simulink model "main2"  (R2024a)
settings: Solver=ode15s  StartTime=0.0  StopTime=2  MaxStep=1e-4  RelTol=1e-3
InitFcn:
  | parametros
values from neighbouring files (symbols this model uses):
  alpha_cu = 3.9 *10^-3    (= 0.0039)    [parametros.m]
  b_l = 0.1    [parametros.m]
  b_m = 1.5 * 10^-5    (= 1.5e-05)    [parametros.m]
  C_ts = 0.818    [parametros.m]
  J_l = (m*l_cm^2 + J_cm) + (m_l * l_l^2)    (= 0.0833)    [parametros.m]
  J_m = 1.4 * 10^-5    (= 1.4e-05)    [parametros.m]
  k_l = m * g * l_cm + m_l * g * l_l    (= 2.4516625)    [parametros.m]
  L_d = 6.6 * 10^-3    (= 0.0066)    [parametros.m]
  L_ls = 0.8 * 10^-3    (= 0.0008)    [parametros.m]
  L_q = 5.8 * 10^-3    (= 0.0058)    [parametros.m]
  lambda_m = 0.016    [parametros.m]
  P_p = 3    [parametros.m]
  r = 120    [parametros.m]
  R_s_40 = 1.02    [parametros.m]
  R_ts_amb = 146.7    [parametros.m]
  Temp_s_ref = 40    [parametros.m]
undefined symbols (not defined in the file or in its folder): K_e_omega, K_e_theta
libraries: simulink x6
(part 1 of 2)
settings Model: Creator=Usuario  LastModifiedBy=Usuario

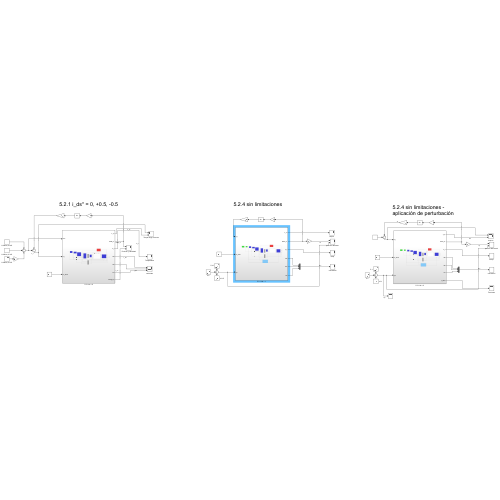
[thumbnail: Simulink's stored preview of the top-level diagram]
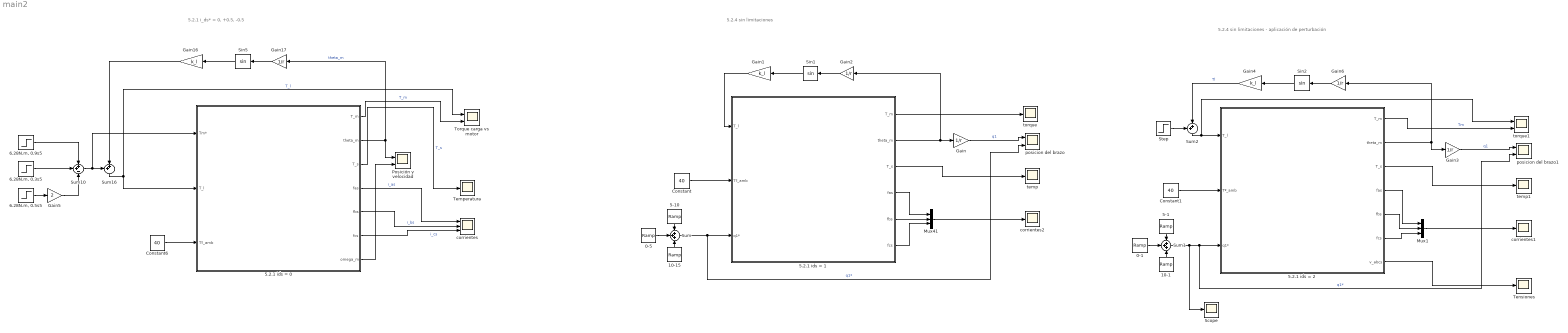
== system main2 ==
  note: 5.2.1 i_ds* = 0, +0.5, -0.5
  note: 5.2.4 sin limitaciones
  note: 5.2.4 sin limitaciones - aplicación de perturbación
  0-1 : simulink/Sources/Ramp  slope=1/5  start=0  InitialOutput=0
  0-5 : simulink/Sources/Ramp  slope=2*pi/5  start=0  InitialOutput=0
  10-1 : simulink/Sources/Ramp  slope=-1/5  start=10  InitialOutput=0
  10-15 : simulink/Sources/Ramp  slope=-2*pi/5  start=10  InitialOutput=0
  5-1 : simulink/Sources/Ramp  slope=-1/5  start=5  InitialOutput=0
  5-10 : simulink/Sources/Ramp  slope=-2*pi/5  start=5  InitialOutput=0
  5.2.1 ids = 0 : Subsystem
  5.2.1 ids = 1 : Subsystem
  5.2.1 ids = 2 : Subsystem
  "6.28N.m, 0.3s5" : Step  Time=0.3  After=6.28  SampleTime=0
  "6.28N.m, 0.5s5" : Step  Time=.5  After=6.28  SampleTime=0
  "6.28N.m, 0.9s5" : Step  Time=.9  After=6.28  SampleTime=0
  Constant : Constant  Value=40
  Constant1 : Constant  Value=40
  Constant6 : Constant  Value=40
  Gain{,2..3,6,17} (5 alike) : Gain  Gain=1/r
  Gain1 : Gain  Gain=k_l
  Gain16 : Gain  Gain=k_l
  Gain4 : Gain  Gain=k_l
  Gain5 : Gain  Gain=2
  Mux1 : Mux  Inputs=3
  Mux41 : Mux  Inputs=3
  Posición y velocidad : Scope  NumInputPorts=2
  Scope : Scope
  Sin1 : Trigonometry
  Sin2 : Trigonometry
  Sin5 : Trigonometry
  Step : Step  Time=7.5  After=2*pi  SampleTime=0
  Sum : Sum  Inputs=+++
  Sum1 : Sum  Inputs=+++
  Sum10 : Sum  Inputs=++-
  Sum16 : Sum  Inputs=++|
  Sum2 : Sum  Inputs=++|
  Temperatura : Scope
  Tensiones : Scope
  Torque carga vs motor : Scope  NumInputPorts=2
  corrientes : Scope  NumInputPorts=3
  corrientes1 : Scope
  corrientes2 : Scope
  posicion del brazo : Scope  NumInputPorts=2
  posicion del brazo1 : Scope  NumInputPorts=2
  temp : Scope
  temp1 : Scope
  torque : Scope
  torque1 : Scope  NumInputPorts=2
  wires:
  5.2.1 ids = 1/6(fcs) -> Mux41/3
  5.2.1 ids = 1/4(fas) -> Mux41/1
  5.2.1 ids = 1/5(fbs) -> Mux41/2
  Mux41/1 -> corrientes2/1
  5.2.1 ids = 1/2("theta_m ") -> Gain/1, Gain2/1
  Sin1/1 -> Gain1/1
  Gain2/1 -> Sin1/1
  Constant/1 -> 5.2.1 ids = 1/2(Tº_amb)
  5.2.1 ids = 1/3(T_s) -> temp/1
  "6.28N.m, 0.3s5"/1 -> Sum10/2
  5.2.1 ids = 0/2("theta_m ") -> Posición y velocidad/1, Gain17/1  "theta_m"
  Constant6/1 -> 5.2.1 ids = 0/3(Tº_amb)
  "6.28N.m, 0.5s5"/1 -> Gain5/1
  Gain5/1 -> Sum10/3
  5.2.1 ids = 0/6(fcs) -> corrientes/3  "i_cs"
  5.2.1 ids = 0/5(fbs) -> corrientes/2  "i_bs"
  5.2.1 ids = 0/1(T_m) -> Torque carga vs motor/2  "T_m"
  5.2.1 ids = 0/4(fas) -> corrientes/1  "i_as"
  Sum16/1 -> 5.2.1 ids = 0/2(T_l), Torque carga vs motor/1  "T_l"
  5.2.1 ids = 0/3(T_s) -> Temperatura/1  "T_s"
  Gain17/1 -> Sin5/1
  "6.28N.m, 0.9s5"/1 -> Sum10/1
  Sin5/1 -> Gain16/1
  5.2.1 ids = 1/1(T_m) -> torque/1
  Gain1/1 -> 5.2.1 ids = 1/1(T_l)
  Sum/1 -> posicion del brazo/2, 5.2.1 ids = 1/3(q1*)  "q1*"
  0-5/1 -> Sum/2
  Gain/1 -> posicion del brazo/1  "q1"
  5-10/1 -> Sum/1
  10-15/1 -> Sum/3
  5-1/1 -> Sum1/1
  Sum1/1 -> Scope/1, posicion del brazo1/2, 5.2.1 ids = 2/3(q1*)  "q1*"
  0-1/1 -> Sum1/2
  5.2.1 ids = 2/1(T_m) -> torque1/2  "Tm"
  Gain3/1 -> posicion del brazo1/1  "q1"
  10-1/1 -> Sum1/3
  Mux1/1 -> corrientes1/1
  5.2.1 ids = 2/3(T_s) -> temp1/1
  5.2.1 ids = 2/6(fcs) -> Mux1/3
  5.2.1 ids = 2/5(fbs) -> Mux1/2
  Constant1/1 -> 5.2.1 ids = 2/2(Tº_amb)
  Gain6/1 -> Sin2/1
  5.2.1 ids = 2/2("theta_m ") -> Gain3/1, Gain6/1
  5.2.1 ids = 2/4(fas) -> Mux1/1
  Sin2/1 -> Gain4/1
  Gain4/1 -> Sum2/2  "Tl"
  Sum2/1 -> torque1/1, 5.2.1 ids = 2/1(T_l)
  Step/1 -> Sum2/1
  5.2.1 ids = 2/7(v_abcs) -> Tensiones/1
  Gain16/1 -> Sum16/2
  Sum10/1 -> 5.2.1 ids = 0/1(Tm*), Sum16/1
  5.2.1 ids = 0/7(omega_m) -> Posición y velocidad/2

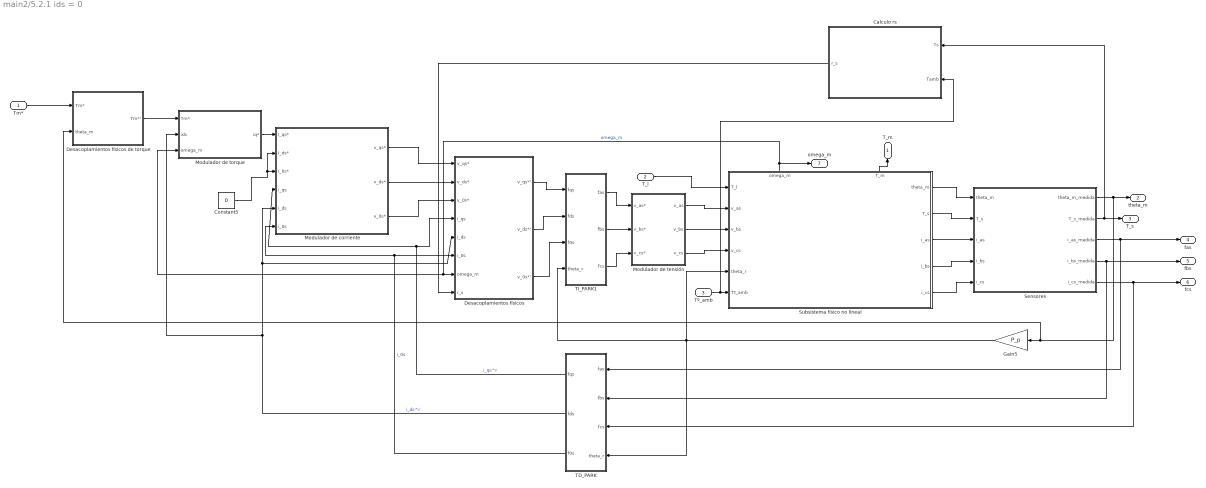
== system main2/5.2.1 ids = 0 ==
  Tm* : Inport
  T_l : Inport  Port=2
  Tº_amb : Inport  Port=3
  Calculo rs : Subsystem
  Constant5 : Constant  Value=0
  Desacoplamientos físicos : Subsystem
  Desacoplamientos físicos de torque : Subsystem
  Gain5 : Gain  Gain=P_p
  Modulador de corriente : Subsystem
  Modulador de tensión : Subsystem
  Modulador de torque : Subsystem
  Sensores : Subsystem
  "Subsistema físico no lineal " : Subsystem
      settings: PortSchema="{\"entries\":[{\"content\":{\"sides\":[{\"content\":{\"connectorIds\":[\"In1\",\"In2\",\"In3\",\"In4\",\"In5\",\"In6\"]},\"type\":\"ConnectorPlacement.EquallySpacedRectSide\",\"uuid\":\"df16c937-5b0d-437b-9581-4e7e4443d731\"},{\"content\":{\"connectorIds\":[\"Out1\",\"Out2\",\"Out3\",\"Out4\",\"Out5\"],\"side\":\"RIGHT\"},\"type\":\"ConnectorPlacement.EquallySpacedRectSide\",\"uuid\":\"58799b56-1bb2-4861-ad63-3fa3f8181ad5\"},{\"content\":{\"connectorIds\":[\"Out6\",\"Out7\"],\"side\":\"TOP\"},\"type\":\"ConnectorPlacement.EquallySpacedRectSide\",\"uuid\":\"9d658df7-49d2-4fa1-a84c-b158d9dac98e\"}]},\"type\":\"ConnectorPlacement.EquallySpacedConnector\",\"uuid\":\"4e139d46-6a94-417e-9cad-9c9676c83a39\"}],\"packageUris\":[\"http://schema.mathworks.com/mf0/Connector/R2020b\"],\"version\":\"1.0\"}"
  TD_PARK : MATLAB Function  TreatAsAtomicUnit=on
  TI_PARK1 : MATLAB Function  TreatAsAtomicUnit=on
  T_m : Outport
  "theta_m " : Outport  Port=2
  T_s : Outport  Port=3
  fas : Outport  Port=4
  fbs : Outport  Port=5
  fcs : Outport  Port=6
  omega_m : Outport  Port=7
  wires:
  Modulador de tensión/1(v_as) -> "Subsistema físico no lineal "/2(v_as)
  TD_PARK/3(f0s) -> Desacoplamientos físicos/6(i_0s), Modulador de corriente/6(i_0s)  "i_0s"
  TI_PARK1/1(fas) -> Modulador de tensión/1(v_as*)
  Sensores/2(T_s_medida) -> T_s/1, Calculo rs/1(Ts)
  Modulador de tensión/2(v_bs) -> "Subsistema físico no lineal "/3(v_bs)
  TD_PARK/1(fqs) -> Modulador de corriente/4(i_qs), Desacoplamientos físicos/4(i_qs)  "i_qs^r"
  Sensores/1(theta_m_medida) -> "theta_m "/1, Desacoplamientos físicos de torque/2(theta_m), Gain5/1
  TI_PARK1/2(fbs) -> Modulador de tensión/2(v_bs*)
  TD_PARK/2(fds) -> Modulador de torque/2(ids), Desacoplamientos físicos/5(i_ds), Modulador de corriente/5(i_ds)  "i_ds^r"
  Desacoplamientos físicos/3(v_0s*') -> TI_PARK1/3(f0s)
  Modulador de tensión/3(v_cs) -> "Subsistema físico no lineal "/4(v_cs)
  "Subsistema físico no lineal "/1(theta_m) -> Sensores/1(theta_m)
  "Subsistema físico no lineal "/2(T_s) -> Sensores/2(T_s)
  Sensores/5(i_cs_medida) -> fcs/1, TD_PARK/3(fcs)
  "Subsistema físico no lineal "/3(i_as) -> Sensores/3(i_as)
  Modulador de torque/1(iq*) -> Modulador de corriente/1(I_qs*)
  Gain5/1 -> "Subsistema físico no lineal "/5(theta_r), TD_PARK/4(theta_r), TI_PARK1/4(theta_r)
  Sensores/4(i_bs_medida) -> fbs/1, TD_PARK/2(fbs)
  "Subsistema físico no lineal "/7(T_m) -> T_m/1
  Modulador de corriente/1(v_qs*) -> Desacoplamientos físicos/1(v_qs*)
  Constant5/1 -> Modulador de corriente/3(I_0s*), Modulador de corriente/2(I_ds*)
  T_l/1 -> "Subsistema físico no lineal "/1(T_l)
  "Subsistema físico no lineal "/4(i_bs) -> Sensores/4(i_bs)
  Modulador de corriente/3(v_0s*) -> Desacoplamientos físicos/3(v_0s*)
  "Subsistema físico no lineal "/6(omega_m) -> omega_m/1, Desacoplamientos físicos/7(omega_m), Modulador de torque/3(omega_m)  "omega_m"
  "Subsistema físico no lineal "/5(i_cs) -> Sensores/5(i_cs)
  Desacoplamientos físicos/1(v_qs*') -> TI_PARK1/1(fqs)
  Sensores/3(i_as_medida) -> TD_PARK/1(fas), fas/1
  TI_PARK1/3(fcs) -> Modulador de tensión/3(v_cs*)
  Tº_amb/1 -> "Subsistema físico no lineal "/6(Tº_amb), Calculo rs/2(Tamb)
  Desacoplamientos físicos/2(v_ds*') -> TI_PARK1/2(fds)
  Modulador de corriente/2(v_ds*) -> Desacoplamientos físicos/2(v_ds*)
  Calculo rs/1(r_s) -> Desacoplamientos físicos/8(r_s)
  Desacoplamientos físicos de torque/1(Tm*') -> Modulador de torque/1(Tm*)
  Tm*/1 -> Desacoplamientos físicos de torque/1(Tm*)

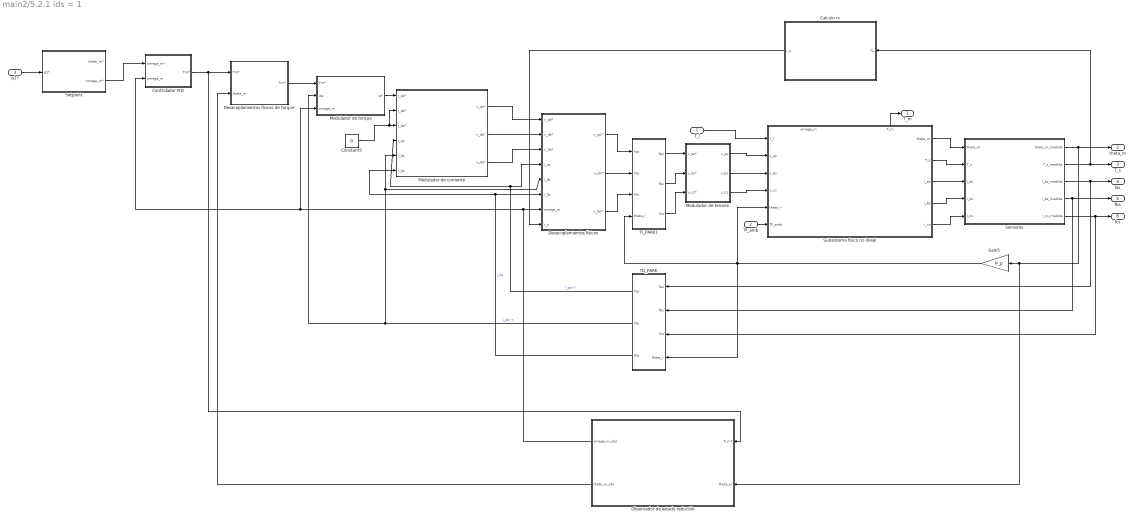
== system main2/5.2.1 ids = 1 ==
  T_l : Inport
  Tº_amb : Inport  Port=2
  q1* : Inport  Port=3
  Calculo rs : Subsystem
  Constant5 : Constant  Value=0
  Controlador PID : Subsystem
  Desacoplamientos físicos : Subsystem
  Desacoplamientos físicos de torque : Subsystem
  Gain5 : Gain  Gain=P_p
  Modulador de corriente : Subsystem
  Modulador de tensión : Subsystem
  Modulador de torque : Subsystem
  Observador de estado reducido : Subsystem
  Sensores : Subsystem
  Setpoint : Subsystem
  "Subsistema físico no lineal " : Subsystem
      settings: PortSchema="{\"entries\":[{\"content\":{\"sides\":[{\"content\":{\"connectorIds\":[\"In1\",\"In2\",\"In3\",\"In4\",\"In5\",\"In6\"]},\"type\":\"ConnectorPlacement.EquallySpacedRectSide\",\"uuid\":\"df16c937-5b0d-437b-9581-4e7e4443d731\"},{\"content\":{\"connectorIds\":[\"Out1\",\"Out2\",\"Out3\",\"Out4\",\"Out5\"],\"side\":\"RIGHT\"},\"type\":\"ConnectorPlacement.EquallySpacedRectSide\",\"uuid\":\"58799b56-1bb2-4861-ad63-3fa3f8181ad5\"},{\"content\":{\"connectorIds\":[\"Out6\",\"Out7\"],\"side\":\"TOP\"},\"type\":\"ConnectorPlacement.EquallySpacedRectSide\",\"uuid\":\"9d658df7-49d2-4fa1-a84c-b158d9dac98e\"}]},\"type\":\"ConnectorPlacement.EquallySpacedConnector\",\"uuid\":\"4e139d46-6a94-417e-9cad-9c9676c83a39\"}],\"packageUris\":[\"http://schema.mathworks.com/mf0/Connector/R2020b\"],\"version\":\"1.0\"}"
  TD_PARK : MATLAB Function  TreatAsAtomicUnit=on
  TI_PARK1 : MATLAB Function  TreatAsAtomicUnit=on
  T_m : Outport
  "theta_m " : Outport  Port=2
  T_s : Outport  Port=3
  fas : Outport  Port=4
  fbs : Outport  Port=5
  fcs : Outport  Port=6
  wires:
  Modulador de tensión/1(v_as) -> "Subsistema físico no lineal "/2(v_as)
  TD_PARK/3(f0s) -> Modulador de corriente/6(i_0s), Desacoplamientos físicos/6(i_0s)  "i_0s"
  TI_PARK1/1(fas) -> Modulador de tensión/1(v_as*)
  Modulador de tensión/2(v_bs) -> "Subsistema físico no lineal "/3(v_bs)
  TD_PARK/1(fqs) -> Modulador de corriente/4(i_qs), Desacoplamientos físicos/4(i_qs)  "i_qs^r"
  Gain5/1 -> "Subsistema físico no lineal "/5(theta_r), TD_PARK/4(theta_r), TI_PARK1/4(theta_r)
  TI_PARK1/2(fbs) -> Modulador de tensión/2(v_bs*)
  TD_PARK/2(fds) -> Modulador de torque/2(ids), Modulador de corriente/5(i_ds), Desacoplamientos físicos/5(i_ds)  "i_ds^r"
  Desacoplamientos físicos/3(v_0s*') -> TI_PARK1/3(f0s)
  Modulador de tensión/3(v_cs) -> "Subsistema físico no lineal "/4(v_cs)
  "Subsistema físico no lineal "/1(theta_m) -> Sensores/1(theta_m)
  "Subsistema físico no lineal "/2(T_s) -> Sensores/2(T_s)
  Sensores/5(i_cs_medida) -> fcs/1, TD_PARK/3(fcs)
  "Subsistema físico no lineal "/3(i_as) -> Sensores/3(i_as)
  Modulador de torque/1(iq*) -> Modulador de corriente/1(I_qs*)
  Sensores/4(i_bs_medida) -> fbs/1, TD_PARK/2(fbs)
  "Subsistema físico no lineal "/7(T_m) -> T_m/1
  Modulador de corriente/1(v_qs*) -> Desacoplamientos físicos/1(v_qs*)
  Constant5/1 -> Modulador de corriente/3(I_0s*), Modulador de corriente/2(I_ds*)
  T_l/1 -> "Subsistema físico no lineal "/1(T_l)
  "Subsistema físico no lineal "/4(i_bs) -> Sensores/4(i_bs)
  Modulador de corriente/3(v_0s*) -> Desacoplamientos físicos/3(v_0s*)
  "Subsistema físico no lineal "/5(i_cs) -> Sensores/5(i_cs)
  Sensores/1(theta_m_medida) -> "theta_m "/1, Observador de estado reducido/2(theta_m), Gain5/1
  Desacoplamientos físicos/1(v_qs*') -> TI_PARK1/1(fqs)
  Sensores/3(i_as_medida) -> TD_PARK/1(fas), fas/1
  TI_PARK1/3(fcs) -> Modulador de tensión/3(v_cs*)
  Desacoplamientos físicos/2(v_ds*') -> TI_PARK1/2(fds)
  Modulador de corriente/2(v_ds*) -> Desacoplamientos físicos/2(v_ds*)
  Setpoint/2(omega_m*) -> Controlador PID/1(omega_m*)
  q1*/1 -> Setpoint/1(q1*)
  Controlador PID/1(Tm*) -> Observador de estado reducido/1(T_m*), Desacoplamientos físicos de torque/1(Tm*)
  Observador de estado reducido/1(omega_m_obs) -> Modulador de torque/3(omega_m), Controlador PID/2(omega_m), Desacoplamientos físicos/7(omega_m)
  Tº_amb/1 -> "Subsistema físico no lineal "/6(Tº_amb)
  Sensores/2(T_s_medida) -> Calculo rs/1(Ts), T_s/1
  Calculo rs/1(r_s) -> Desacoplamientos físicos/8(r_s)
  Desacoplamientos físicos de torque/1(Tm*') -> Modulador de torque/1(Tm*)
  Observador de estado reducido/2(theta_m_obs) -> Desacoplamientos físicos de torque/2(theta_m)

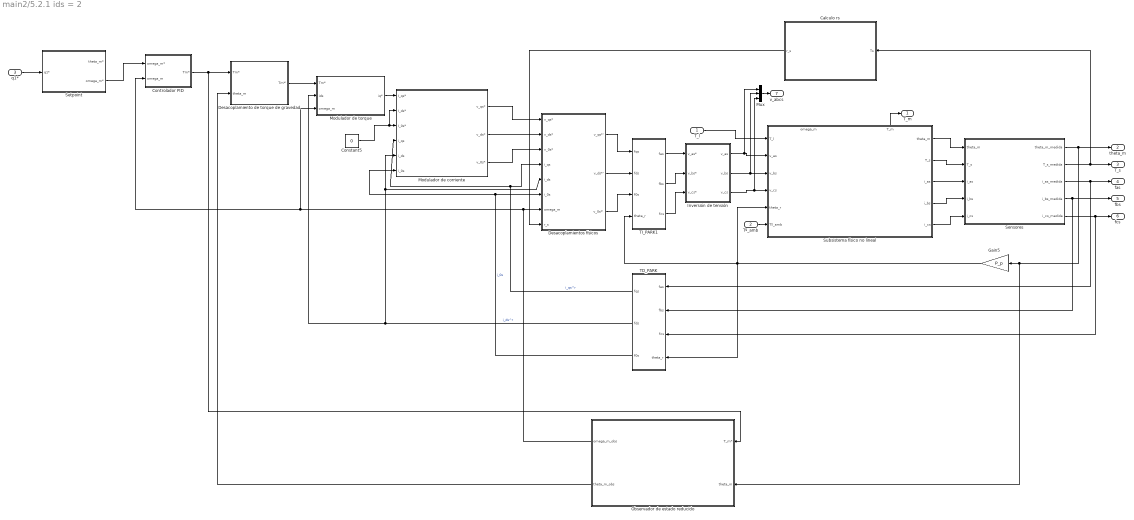
== system main2/5.2.1 ids = 2 ==
  T_l : Inport
  Tº_amb : Inport  Port=2
  q1* : Inport  Port=3
  Calculo rs : Subsystem
  Constant5 : Constant  Value=0
  Controlador PID : Subsystem
  Desacoplamiento de torque de gravedad : Subsystem
  Desacoplamientos físicos : Subsystem
  Gain5 : Gain  Gain=P_p
  Inversión de tensión : Subsystem
  Modulador de corriente : Subsystem
  Modulador de torque : Subsystem
  Mux : Mux  Inputs=3
  Observador de estado reducido : Subsystem
  Sensores : Subsystem
  Setpoint : Subsystem
  "Subsistema físico no lineal " : Subsystem
      settings: PortSchema="{\"entries\":[{\"content\":{\"sides\":[{\"content\":{\"connectorIds\":[\"In1\",\"In2\",\"In3\",\"In4\",\"In5\",\"In6\"]},\"type\":\"ConnectorPlacement.EquallySpacedRectSide\",\"uuid\":\"df16c937-5b0d-437b-9581-4e7e4443d731\"},{\"content\":{\"connectorIds\":[\"Out1\",\"Out2\",\"Out3\",\"Out4\",\"Out5\"],\"side\":\"RIGHT\"},\"type\":\"ConnectorPlacement.EquallySpacedRectSide\",\"uuid\":\"58799b56-1bb2-4861-ad63-3fa3f8181ad5\"},{\"content\":{\"connectorIds\":[\"Out6\",\"Out7\"],\"side\":\"TOP\"},\"type\":\"ConnectorPlacement.EquallySpacedRectSide\",\"uuid\":\"9d658df7-49d2-4fa1-a84c-b158d9dac98e\"}]},\"type\":\"ConnectorPlacement.EquallySpacedConnector\",\"uuid\":\"4e139d46-6a94-417e-9cad-9c9676c83a39\"}],\"packageUris\":[\"http://schema.mathworks.com/mf0/Connector/R2020b\"],\"version\":\"1.0\"}"
  TD_PARK : MATLAB Function  TreatAsAtomicUnit=on
  TI_PARK1 : MATLAB Function  TreatAsAtomicUnit=on
  T_m : Outport
  "theta_m " : Outport  Port=2
  T_s : Outport  Port=3
  fas : Outport  Port=4
  fbs : Outport  Port=5
  fcs : Outport  Port=6
  v_abcs : Outport  Port=7
  wires:
  Inversión de tensión/1(v_as) -> Mux/1, "Subsistema físico no lineal "/2(v_as)
  TD_PARK/3(f0s) -> Modulador de corriente/6(i_0s), Desacoplamientos físicos/6(i_0s)  "i_0s"
  TI_PARK1/1(fas) -> Inversión de tensión/1(v_as*)
  Inversión de tensión/2(v_bs) -> Mux/2, "Subsistema físico no lineal "/3(v_bs)
  TD_PARK/1(fqs) -> Modulador de corriente/4(i_qs), Desacoplamientos físicos/4(i_qs)  "i_qs^r"
  Gain5/1 -> "Subsistema físico no lineal "/5(theta_r), TD_PARK/4(theta_r), TI_PARK1/4(theta_r)
  TI_PARK1/2(fbs) -> Inversión de tensión/2(v_bs*)
  TD_PARK/2(fds) -> Modulador de torque/2(ids), Modulador de corriente/5(i_ds), Desacoplamientos físicos/5(i_ds)  "i_ds^r"
  Desacoplamientos físicos/3(v_0s*') -> TI_PARK1/3(f0s)
  Inversión de tensión/3(v_cs) -> Mux/3, "Subsistema físico no lineal "/4(v_cs)
  "Subsistema físico no lineal "/1(theta_m) -> Sensores/1(theta_m)
  "Subsistema físico no lineal "/2(T_s) -> Sensores/2(T_s)
  Sensores/5(i_cs_medida) -> fcs/1, TD_PARK/3(fcs)
  "Subsistema físico no lineal "/3(i_as) -> Sensores/3(i_as)
  Modulador de torque/1(iq*) -> Modulador de corriente/1(I_qs*)
  Sensores/4(i_bs_medida) -> fbs/1, TD_PARK/2(fbs)
  "Subsistema físico no lineal "/7(T_m) -> T_m/1
  Modulador de corriente/1(v_qs*) -> Desacoplamientos físicos/1(v_qs*)
  Constant5/1 -> Modulador de corriente/3(I_0s*), Modulador de corriente/2(I_ds*)
  T_l/1 -> "Subsistema físico no lineal "/1(T_l)
  "Subsistema físico no lineal "/4(i_bs) -> Sensores/4(i_bs)
  Modulador de corriente/3(v_0s*) -> Desacoplamientos físicos/3(v_0s*)
  "Subsistema físico no lineal "/5(i_cs) -> Sensores/5(i_cs)
  Sensores/1(theta_m_medida) -> "theta_m "/1, Observador de estado reducido/2(theta_m), Gain5/1
  Desacoplamientos físicos/1(v_qs*') -> TI_PARK1/1(fqs)
  Sensores/3(i_as_medida) -> TD_PARK/1(fas), fas/1
  TI_PARK1/3(fcs) -> Inversión de tensión/3(v_cs*)
  Desacoplamientos físicos/2(v_ds*') -> TI_PARK1/2(fds)
  Modulador de corriente/2(v_ds*) -> Desacoplamientos físicos/2(v_ds*)
  Setpoint/2(omega_m*) -> Controlador PID/1(omega_m*)
  q1*/1 -> Setpoint/1(q1*)
  Controlador PID/1(Tm*) -> Observador de estado reducido/1(T_m*), Desacoplamiento de torque de gravedad/1(Tm*)
  Observador de estado reducido/1(omega_m_obs) -> Modulador de torque/3(omega_m), Controlador PID/2(omega_m), Desacoplamientos físicos/7(omega_m)
  Tº_amb/1 -> "Subsistema físico no lineal "/6(Tº_amb)
  Sensores/2(T_s_medida) -> Calculo rs/1(Ts), T_s/1
  Calculo rs/1(r_s) -> Desacoplamientos físicos/8(r_s)
  Desacoplamiento de torque de gravedad/1(Tm*') -> Modulador de torque/1(Tm*)
  Observador de estado reducido/2(theta_m_obs) -> Desacoplamiento de torque de gravedad/2(theta_m)
  Mux/1 -> v_abcs/1

== system main2/5.2.1 ids = 0/Calculo rs ==
  Ts : Inport
  Tamb : Inport  Port=2
  Constant : Constant
  Gain : Gain  Gain=alpha_cu
  Gain1 : Gain  Gain=R_s_40
  Sum : Sum  Inputs=|++
  Sum1 : Sum  Inputs=|-+
  r_s : Outport
  wires:
  Constant/1 -> Sum/1
  Gain/1 -> Sum/2
  Ts/1 -> Sum1/2
  Tamb/1 -> Sum1/1
  Sum1/1 -> Gain/1
  Sum/1 -> Gain1/1
  Gain1/1 -> r_s/1

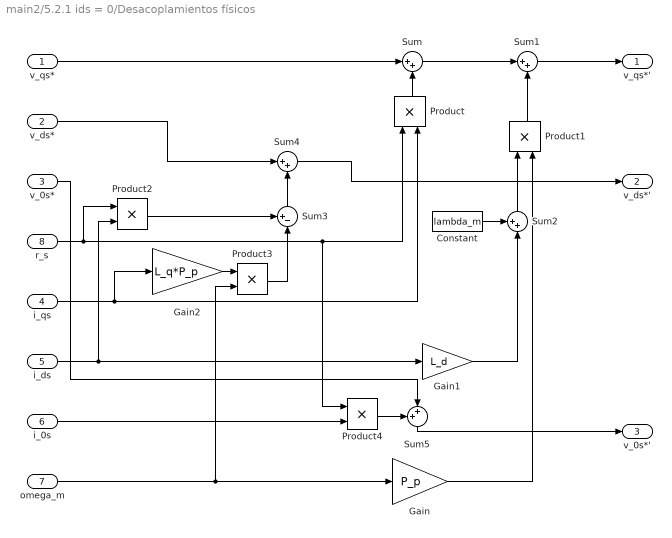
== system main2/5.2.1 ids = 0/Desacoplamientos físicos ==
  v_qs* : Inport
  v_ds* : Inport  Port=2
  v_0s* : Inport  Port=3
  i_qs : Inport  Port=4
  i_ds : Inport  Port=5
  i_0s : Inport  Port=6
  omega_m : Inport  Port=7
  r_s : Inport  Port=8
  Constant : Constant  Value=lambda_m
  Gain : Gain  Gain=P_p
  Gain1 : Gain  Gain=L_d
  Gain2 : Gain  Gain=L_q*P_p
  Product{,1..4} (5 alike) : Product
  Sum : Sum  Inputs=|++
  Sum1 : Sum  Inputs=|++
  Sum2 : Sum  Inputs=++|
  Sum3 : Sum  Inputs=+-|
  Sum4 : Sum  Inputs=|++
  Sum5 : Sum  Inputs=++|
  v_qs*' : Outport
  v_ds*' : Outport  Port=2
  v_0s*' : Outport  Port=3
  wires:
  Product/1 -> Sum/2
  r_s/1 -> Product4/1, Product/1, Product2/1
  i_qs/1 -> Product/2, Gain2/1
  v_qs*/1 -> Sum/1
  Sum/1 -> Sum1/1
  omega_m/1 -> Product3/2, Gain/1
  Product1/1 -> Sum1/2
  Gain/1 -> Product1/2
  i_ds/1 -> Gain1/1, Product2/2
  Gain1/1 -> Sum2/2
  Constant/1 -> Sum2/1
  Sum2/1 -> Product1/1
  Sum1/1 -> v_qs*'/1
  Product2/1 -> Sum3/1
  Gain2/1 -> Product3/1
  Product3/1 -> Sum3/2
  Sum3/1 -> Sum4/2
  v_ds*/1 -> Sum4/1
  Sum4/1 -> v_ds*'/1
  i_0s/1 -> Product4/2
  Product4/1 -> Sum5/1
  v_0s*/1 -> Sum5/2
  Sum5/1 -> v_0s*'/1

== system main2/5.2.1 ids = 0/Desacoplamientos físicos de torque ==
  Tm* : Inport
  theta_m : Inport  Port=2
  Gain : Gain  Gain=k_l
  Gain1 : Gain  Gain=1/r
  Sin : Trigonometry
  Sum : Sum  Inputs=|++
  Tm*' : Outport
  wires:
  Tm*/1 -> Sum/1
  theta_m/1 -> Gain1/1
  Sin/1 -> Gain/1
  Sum/1 -> Tm*'/1
  Gain1/1 -> Sin/1
  Gain/1 -> Sum/2

== system main2/5.2.1 ids = 0/Modulador de corriente ==
  I_qs* : Inport
  I_ds* : Inport  Port=2
  I_0s* : Inport  Port=3
  i_qs : Inport  Port=4
  i_ds : Inport  Port=5
  i_0s : Inport  Port=6
  Gain : Gain  Gain=5000*L_q
  Gain1 : Gain  Gain=5000*L_d
  Gain2 : Gain  Gain=5000*L_ls
  Sum : Sum  Inputs=+-
  Sum1 : Sum  Inputs=+-
  Sum2 : Sum  Inputs=+-
  v_qs* : Outport
  v_ds* : Outport  Port=2
  v_0s* : Outport  Port=3
  wires:
  Sum2/1 -> Gain2/1
  Sum1/1 -> Gain1/1
  Sum/1 -> Gain/1
  I_qs*/1 -> Sum/1
  i_qs/1 -> Sum/2
  I_ds*/1 -> Sum1/1
  i_ds/1 -> Sum1/2
  I_0s*/1 -> Sum2/1
  i_0s/1 -> Sum2/2
  Gain/1 -> v_qs*/1
  Gain2/1 -> v_0s*/1
  Gain1/1 -> v_ds*/1

== system main2/5.2.1 ids = 0/Modulador de tensión ==
  v_as* : Inport
  v_bs* : Inport  Port=2
  v_cs* : Inport  Port=3
  Gain : Gain
  Gain1 : Gain
  Gain2 : Gain
  v_as : Outport
  v_bs : Outport  Port=2
  v_cs : Outport  Port=3
  wires:
  v_as*/1 -> Gain/1
  Gain/1 -> v_as/1
  v_bs*/1 -> Gain1/1
  Gain1/1 -> v_bs/1
  v_cs*/1 -> Gain2/1
  Gain2/1 -> v_cs/1

== system main2/5.2.1 ids = 0/Modulador de torque ==
  Tm* : Inport
  ids : Inport  Port=2
  omega_m : Inport  Port=3
  Constant : Constant  Value=lambda_m
  Divide : Product  Inputs=/*
  Gain : Gain  Gain=b_m + b_l/r^2
  Gain1 : Gain  Gain=2/(3*P_p)
  Gain2 : Gain  Gain=L_d-L_q
  Sum : Sum  Inputs=|++
  Sum1 : Sum  Inputs=++|
  iq* : Outport
  wires:
  omega_m/1 -> Gain/1
  Sum/1 -> Gain1/1
  ids/1 -> Gain2/1
  Gain2/1 -> Sum1/1
  Constant/1 -> Sum1/2
  Sum1/1 -> Divide/1
  Gain/1 -> Sum/2
  Tm*/1 -> Sum/1
  Gain1/1 -> Divide/2
  Divide/1 -> iq*/1

== system main2/5.2.1 ids = 0/Sensores ==
  theta_m : Inport
  T_s : Inport  Port=2
  i_as : Inport  Port=3
  i_bs : Inport  Port=4
  i_cs : Inport  Port=5
  Gain{,1..4} (5 alike) : Gain
  theta_m_medida : Outport
  T_s_medida : Outport  Port=2
  i_as_medida : Outport  Port=3
  i_bs_medida : Outport  Port=4
  i_cs_medida : Outport  Port=5
  wires:
  theta_m/1 -> Gain/1
  T_s/1 -> Gain1/1
  i_as/1 -> Gain2/1
  Gain/1 -> theta_m_medida/1
  Gain1/1 -> T_s_medida/1
  Gain2/1 -> i_as_medida/1
  Gain3/1 -> i_bs_medida/1
  i_bs/1 -> Gain3/1
  i_cs/1 -> Gain4/1
  Gain4/1 -> i_cs_medida/1

== system main2/5.2.1 ids = 0/Subsistema físico no lineal  ==
  T_l : Inport
  v_as : Inport  Port=2
  v_bs : Inport  Port=3
  v_cs : Inport  Port=4
  theta_r : Inport  Port=5
  Tº_amb : Inport  Port=6
  Subsistema electromagnético : Subsystem
  Subsistema mecánico completo : Subsystem
  Subsistema térmico : Subsystem
  TD_PARK : MATLAB Function  TreatAsAtomicUnit=on
  TI_PARK : MATLAB Function  TreatAsAtomicUnit=on
  theta_m : Outport
  T_s : Outport  Port=2
  i_as : Outport  Port=3
  i_bs : Outport  Port=4
  i_cs : Outport  Port=5
  omega_m : Outport  Port=6
  T_m : Outport  Port=7
  wires:
  theta_r/1 -> TI_PARK/4(theta_r), TD_PARK/4(theta_r)
  TI_PARK/2(fbs) -> i_bs/1
  v_cs/1 -> TD_PARK/3(fcs)
  v_as/1 -> TD_PARK/1(fas)
  TI_PARK/3(fcs) -> i_cs/1
  v_bs/1 -> TD_PARK/2(fbs)
  TI_PARK/1(fas) -> i_as/1
  TD_PARK/1(fqs) -> Subsistema electromagnético/1(v_qs^r)
  TD_PARK/2(fds) -> Subsistema electromagnético/2(v_ds^r)
  TD_PARK/3(f0s) -> Subsistema electromagnético/3(v_0s^r)
  Subsistema mecánico completo/2(omega_m(t)) -> Subsistema electromagnético/4(omega_m), omega_m/1
  Subsistema térmico/2(r_s) -> Subsistema electromagnético/5(r_s)
  Subsistema electromagnético/2(i_ds^r) -> Subsistema térmico/2(i_ds^r), TI_PARK/2(fds)
  Subsistema electromagnético/3(i_qs^r) -> Subsistema térmico/1(i_qs^r), TI_PARK/1(fqs)
  Subsistema electromagnético/1(i_0s^r) -> Subsistema térmico/3(i_0s^r), TI_PARK/3(f0s)
  Subsistema electromagnético/4(T_m) -> Subsistema mecánico completo/1(T_m), T_m/1
  T_l/1 -> Subsistema mecánico completo/2(T_l)
  Tº_amb/1 -> Subsistema térmico/4(Tº_amb)
  Subsistema térmico/1(T_s) -> T_s/1
  Subsistema mecánico completo/1(theta_m(t)) -> theta_m/1

== system main2/5.2.1 ids = 1/Calculo rs ==
  Ts : Inport
  Constant : Constant
  Constant1 : Constant  Value=Temp_s_ref
  Gain : Gain  Gain=alpha_cu
  Gain1 : Gain  Gain=R_s_40
  Sum : Sum  Inputs=|++
  Sum1 : Sum  Inputs=|-+
  r_s : Outport
  wires:
  Constant/1 -> Sum/1
  Gain/1 -> Sum/2
  Ts/1 -> Sum1/2
  Constant1/1 -> Sum1/1
  Sum1/1 -> Gain/1
  Sum/1 -> Gain1/1
  Gain1/1 -> r_s/1

== system main2/5.2.1 ids = 1/Controlador PID ==
  note: ba: Proporcional al error de velocidad
  note: Ksa: Proporcional a la integral al error de velocidad
  note: Ksia: Porporcional a la doble Integral al error de velocidad
  omega_m* : Inport
  omega_m : Inport  Port=2
  Gain : Gain  Gain=10137.6
  Gain1 : Gain  Gain=31.68
  Gain2 : Gain  Gain=0.0396
  Integrator : Integrator
  Integrator1 : Integrator
  Sum : Sum  Inputs=|+-
  Sum1 : Sum  Inputs=+++
  Tm* : Outport
  wires:
  omega_m*/1 -> Sum/1
  omega_m/1 -> Sum/2
  Sum/1 -> Integrator/1, Gain/1
  Integrator/1 -> Integrator1/1, Gain1/1
  Gain/1 -> Sum1/3
  Sum1/1 -> Tm*/1
  Gain1/1 -> Sum1/2
  Integrator1/1 -> Gain2/1
  Gain2/1 -> Sum1/1

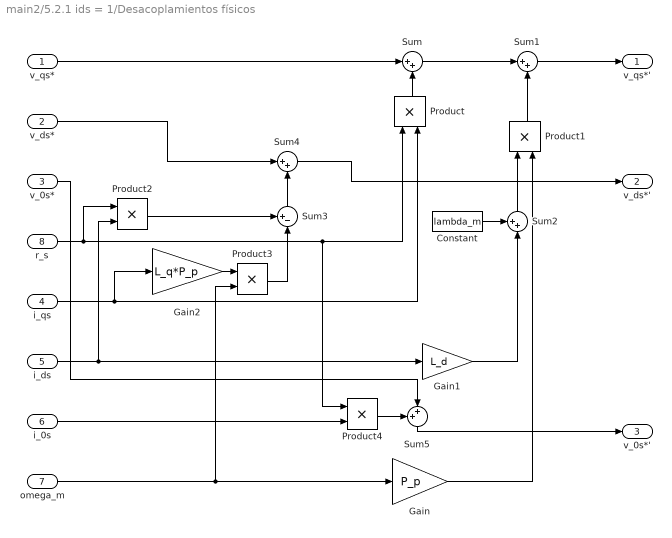
== system main2/5.2.1 ids = 1/Desacoplamientos físicos ==
  v_qs* : Inport
  v_ds* : Inport  Port=2
  v_0s* : Inport  Port=3
  i_qs : Inport  Port=4
  i_ds : Inport  Port=5
  i_0s : Inport  Port=6
  omega_m : Inport  Port=7
  r_s : Inport  Port=8
  Constant : Constant  Value=lambda_m
  Gain : Gain  Gain=P_p
  Gain1 : Gain  Gain=L_d
  Gain2 : Gain  Gain=L_q*P_p
  Product{,1..4} (5 alike) : Product
  Sum : Sum  Inputs=|++
  Sum1 : Sum  Inputs=|++
  Sum2 : Sum  Inputs=++|
  Sum3 : Sum  Inputs=+-|
  Sum4 : Sum  Inputs=|++
  Sum5 : Sum  Inputs=++|
  v_qs*' : Outport
  v_ds*' : Outport  Port=2
  v_0s*' : Outport  Port=3
  wires:
  Product/1 -> Sum/2
  r_s/1 -> Product4/1, Product/1, Product2/1
  i_qs/1 -> Product/2, Gain2/1
  v_qs*/1 -> Sum/1
  Sum/1 -> Sum1/1
  omega_m/1 -> Product3/2, Gain/1
  Product1/1 -> Sum1/2
  Gain/1 -> Product1/2
  i_ds/1 -> Gain1/1, Product2/2
  Gain1/1 -> Sum2/2
  Constant/1 -> Sum2/1
  Sum2/1 -> Product1/1
  Sum1/1 -> v_qs*'/1
  Product2/1 -> Sum3/1
  Gain2/1 -> Product3/1
  Product3/1 -> Sum3/2
  Sum3/1 -> Sum4/2
  v_ds*/1 -> Sum4/1
  Sum4/1 -> v_ds*'/1
  i_0s/1 -> Product4/2
  Product4/1 -> Sum5/1
  v_0s*/1 -> Sum5/2
  Sum5/1 -> v_0s*'/1

== system main2/5.2.1 ids = 1/Desacoplamientos físicos de torque ==
  Tm* : Inport
  theta_m : Inport  Port=2
  Gain : Gain  Gain=k_l
  Gain1 : Gain  Gain=1/r
  Sin : Trigonometry
  Sum : Sum  Inputs=|++
  Tm*' : Outport
  wires:
  Tm*/1 -> Sum/1
  Sin/1 -> Gain/1
  Sum/1 -> Tm*'/1
  Gain1/1 -> Sin/1
  theta_m/1 -> Gain1/1
  Gain/1 -> Sum/2

== system main2/5.2.1 ids = 1/Modulador de corriente ==
  I_qs* : Inport
  I_ds* : Inport  Port=2
  I_0s* : Inport  Port=3
  i_qs : Inport  Port=4
  i_ds : Inport  Port=5
  i_0s : Inport  Port=6
  Gain : Gain  Gain=5000*L_q
  Gain1 : Gain  Gain=5000*L_d
  Gain2 : Gain  Gain=5000*L_ls
  Sum : Sum  Inputs=+-
  Sum1 : Sum  Inputs=+-
  Sum2 : Sum  Inputs=+-
  v_qs* : Outport
  v_ds* : Outport  Port=2
  v_0s* : Outport  Port=3
  wires:
  Sum2/1 -> Gain2/1
  Sum1/1 -> Gain1/1
  Sum/1 -> Gain/1
  I_qs*/1 -> Sum/1
  i_qs/1 -> Sum/2
  I_ds*/1 -> Sum1/1
  i_ds/1 -> Sum1/2
  I_0s*/1 -> Sum2/1
  i_0s/1 -> Sum2/2
  Gain/1 -> v_qs*/1
  Gain2/1 -> v_0s*/1
  Gain1/1 -> v_ds*/1

== system main2/5.2.1 ids = 1/Modulador de tensión ==
  v_as* : Inport
  v_bs* : Inport  Port=2
  v_cs* : Inport  Port=3
  Gain : Gain
  Gain1 : Gain
  Gain2 : Gain
  v_as : Outport
  v_bs : Outport  Port=2
  v_cs : Outport  Port=3
  wires:
  v_as*/1 -> Gain/1
  Gain/1 -> v_as/1
  v_bs*/1 -> Gain1/1
  Gain1/1 -> v_bs/1
  v_cs*/1 -> Gain2/1
  Gain2/1 -> v_cs/1

== system main2/5.2.1 ids = 1/Modulador de torque ==
  Tm* : Inport
  ids : Inport  Port=2
  omega_m : Inport  Port=3
  Constant : Constant  Value=lambda_m
  Divide : Product  Inputs=/*
  Gain : Gain  Gain=b_m + b_l/r^2
  Gain1 : Gain  Gain=2/(3*P_p)
  Gain2 : Gain  Gain=L_d-L_q
  Sum : Sum  Inputs=|++
  Sum1 : Sum  Inputs=++|
  iq* : Outport
  wires:
  omega_m/1 -> Gain/1
  Sum/1 -> Gain1/1
  ids/1 -> Gain2/1
  Gain2/1 -> Sum1/1
  Constant/1 -> Sum1/2
  Sum1/1 -> Divide/1
  Gain/1 -> Sum/2
  Tm*/1 -> Sum/1
  Gain1/1 -> Divide/2
  Divide/1 -> iq*/1

== system main2/5.2.1 ids = 1/Observador de estado reducido ==
  T_m* : Inport
  theta_m : Inport  Port=2
  Gain : Gain  Gain=1/(J_m+(J_l/r^2))
  Gain1 : Gain  Gain=K_e_theta
  Gain2 : Gain  Gain=K_e_omega
  Integrator : Integrator
  Integrator1 : Integrator
  Sum : Sum  Inputs=|++
  Sum1 : Sum  Inputs=|++
  Sum2 : Sum  Inputs=|-+
  omega_m_obs : Outport
  theta_m_obs : Outport  Port=2
  wires:
  T_m*/1 -> Gain/1
  Gain/1 -> Sum/1
  Sum/1 -> Integrator/1
  Integrator1/1 -> theta_m_obs/1, Sum2/1
  Integrator/1 -> Sum1/1
  Sum1/1 -> omega_m_obs/1, Integrator1/1
  theta_m/1 -> Sum2/2
  Gain1/1 -> Sum1/2
  Sum2/1 -> Gain2/1, Gain1/1
  Gain2/1 -> Sum/2

== system main2/5.2.1 ids = 1/Sensores ==
  theta_m : Inport
  T_s : Inport  Port=2
  i_as : Inport  Port=3
  i_bs : Inport  Port=4
  i_cs : Inport  Port=5
  Gain{,1..4} (5 alike) : Gain
  theta_m_medida : Outport
  T_s_medida : Outport  Port=2
  i_as_medida : Outport  Port=3
  i_bs_medida : Outport  Port=4
  i_cs_medida : Outport  Port=5
  wires:
  theta_m/1 -> Gain/1
  T_s/1 -> Gain1/1
  i_as/1 -> Gain2/1
  Gain/1 -> theta_m_medida/1
  Gain1/1 -> T_s_medida/1
  Gain2/1 -> i_as_medida/1
  Gain3/1 -> i_bs_medida/1
  i_bs/1 -> Gain3/1
  i_cs/1 -> Gain4/1
  Gain4/1 -> i_cs_medida/1

== system main2/5.2.1 ids = 1/Setpoint ==
  q1* : Inport
  Derivative : Derivative
  Gain : Gain  Gain=r
  theta_m* : Outport
  omega_m* : Outport  Port=2
  wires:
  q1*/1 -> Gain/1
  Gain/1 -> Derivative/1, theta_m*/1
  Derivative/1 -> omega_m*/1

== system main2/5.2.1 ids = 1/Subsistema físico no lineal  ==
  T_l : Inport
  v_as : Inport  Port=2
  v_bs : Inport  Port=3
  v_cs : Inport  Port=4
  theta_r : Inport  Port=5
  Tº_amb : Inport  Port=6
  Subsistema electromagnético : Subsystem
  Subsistema mecánico completo : Subsystem
  Subsistema térmico : Subsystem
  TD_PARK : MATLAB Function  TreatAsAtomicUnit=on
  TI_PARK : MATLAB Function  TreatAsAtomicUnit=on
  theta_m : Outport
  T_s : Outport  Port=2
  i_as : Outport  Port=3
  i_bs : Outport  Port=4
  i_cs : Outport  Port=5
  omega_m : Outport  Port=6
  T_m : Outport  Port=7
  wires:
  theta_r/1 -> TI_PARK/4(theta_r), TD_PARK/4(theta_r)
  TI_PARK/2(fbs) -> i_bs/1
  v_cs/1 -> TD_PARK/3(fcs)
  v_as/1 -> TD_PARK/1(fas)
  TI_PARK/3(fcs) -> i_cs/1
  v_bs/1 -> TD_PARK/2(fbs)
  TI_PARK/1(fas) -> i_as/1
  TD_PARK/1(fqs) -> Subsistema electromagnético/1(v_qs^r)
  TD_PARK/2(fds) -> Subsistema electromagnético/2(v_ds^r)
  TD_PARK/3(f0s) -> Subsistema electromagnético/3(v_0s^r)
  Subsistema mecánico completo/2(omega_m(t)) -> Subsistema electromagnético/4(omega_m), omega_m/1
  Subsistema térmico/2(r_s) -> Subsistema electromagnético/5(r_s)
  Subsistema electromagnético/2(i_ds^r) -> Subsistema térmico/2(i_ds^r), TI_PARK/2(fds)
  Subsistema electromagnético/3(i_qs^r) -> Subsistema térmico/1(i_qs^r), TI_PARK/1(fqs)
  Subsistema electromagnético/1(i_0s^r) -> Subsistema térmico/3(i_0s^r), TI_PARK/3(f0s)
  Subsistema electromagnético/4(T_m) -> Subsistema mecánico completo/1(T_m), T_m/1
  T_l/1 -> Subsistema mecánico completo/2(T_l)
  Tº_amb/1 -> Subsistema térmico/4(Tº_amb)
  Subsistema térmico/1(T_s) -> T_s/1
  Subsistema mecánico completo/1(theta_m(t)) -> theta_m/1

== system main2/5.2.1 ids = 2/Calculo rs ==
  Ts : Inport
  Constant : Constant
  Constant1 : Constant  Value=Temp_s_ref
  Gain : Gain  Gain=alpha_cu
  Gain1 : Gain  Gain=R_s_40
  Sum : Sum  Inputs=|++
  Sum1 : Sum  Inputs=|-+
  r_s : Outport
  wires:
  Constant/1 -> Sum/1
  Gain/1 -> Sum/2
  Ts/1 -> Sum1/2
  Constant1/1 -> Sum1/1
  Sum1/1 -> Gain/1
  Sum/1 -> Gain1/1
  Gain1/1 -> r_s/1

== system main2/5.2.1 ids = 2/Controlador PID ==
  note: ba: Proporcional al error de velocidad
  note: Ksa: Proporcional a la integral al error de velocidad
  note: Ksia: Porporcional a la doble Integral al error de velocidad
  omega_m* : Inport
  omega_m : Inport  Port=2
  Gain : Gain  Gain=10137.6
  Gain1 : Gain  Gain=31.68
  Gain2 : Gain  Gain=0.0396
  Integrator : Integrator
  Integrator1 : Integrator
  Sum : Sum  Inputs=|+-
  Sum1 : Sum  Inputs=+++
  Tm* : Outport
  wires:
  omega_m*/1 -> Sum/1
  omega_m/1 -> Sum/2
  Sum/1 -> Integrator/1, Gain/1
  Integrator/1 -> Integrator1/1, Gain1/1
  Gain/1 -> Sum1/3
  Sum1/1 -> Tm*/1
  Gain1/1 -> Sum1/2
  Integrator1/1 -> Gain2/1
  Gain2/1 -> Sum1/1

== system main2/5.2.1 ids = 2/Desacoplamiento de torque de gravedad ==
  Tm* : Inport
  theta_m : Inport  Port=2
  Gain : Gain  Gain=k_l
  Gain1 : Gain  Gain=1/r
  Sin : Trigonometry
  Sum : Sum  Inputs=|++
  Tm*' : Outport
  wires:
  Tm*/1 -> Sum/1
  Sin/1 -> Gain/1
  Sum/1 -> Tm*'/1
  Gain1/1 -> Sin/1
  theta_m/1 -> Gain1/1
  Gain/1 -> Sum/2

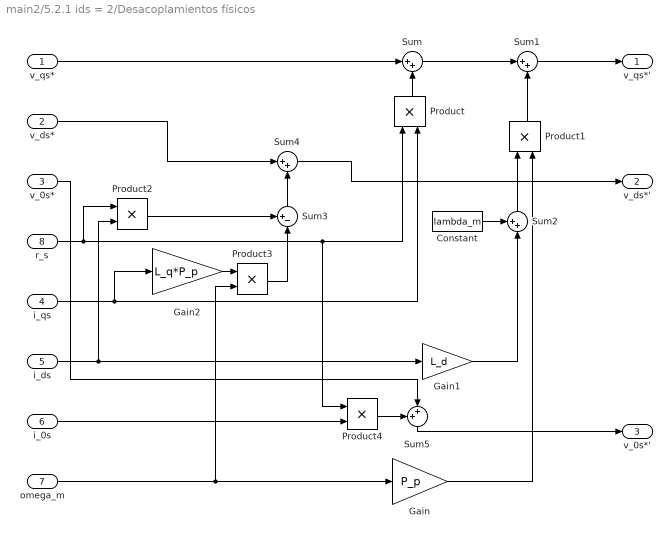
== system main2/5.2.1 ids = 2/Desacoplamientos físicos ==
  v_qs* : Inport
  v_ds* : Inport  Port=2
  v_0s* : Inport  Port=3
  i_qs : Inport  Port=4
  i_ds : Inport  Port=5
  i_0s : Inport  Port=6
  omega_m : Inport  Port=7
  r_s : Inport  Port=8
  Constant : Constant  Value=lambda_m
  Gain : Gain  Gain=P_p
  Gain1 : Gain  Gain=L_d
  Gain2 : Gain  Gain=L_q*P_p
  Product{,1..4} (5 alike) : Product
  Sum : Sum  Inputs=|++
  Sum1 : Sum  Inputs=|++
  Sum2 : Sum  Inputs=++|
  Sum3 : Sum  Inputs=+-|
  Sum4 : Sum  Inputs=|++
  Sum5 : Sum  Inputs=++|
  v_qs*' : Outport
  v_ds*' : Outport  Port=2
  v_0s*' : Outport  Port=3
  wires:
  Product/1 -> Sum/2
  r_s/1 -> Product4/1, Product/1, Product2/1
  i_qs/1 -> Product/2, Gain2/1
  v_qs*/1 -> Sum/1
  Sum/1 -> Sum1/1
  omega_m/1 -> Product3/2, Gain/1
  Product1/1 -> Sum1/2
  Gain/1 -> Product1/2
  i_ds/1 -> Gain1/1, Product2/2
  Gain1/1 -> Sum2/2
  Constant/1 -> Sum2/1
  Sum2/1 -> Product1/1
  Sum1/1 -> v_qs*'/1
  Product2/1 -> Sum3/1
  Gain2/1 -> Product3/1
  Product3/1 -> Sum3/2
  Sum3/1 -> Sum4/2
  v_ds*/1 -> Sum4/1
  Sum4/1 -> v_ds*'/1
  i_0s/1 -> Product4/2
  Product4/1 -> Sum5/1
  v_0s*/1 -> Sum5/2
  Sum5/1 -> v_0s*'/1

== system main2/5.2.1 ids = 2/Inversión de tensión ==
  v_as* : Inport
  v_bs* : Inport  Port=2
  v_cs* : Inport  Port=3
  Gain : Gain
  Gain1 : Gain
  Gain2 : Gain
  Saturation : Saturate  Commented=on  UpperLimit=20  LowerLimit=-20
  Saturation1 : Saturate  Commented=on  UpperLimit=20  LowerLimit=-20
  Saturation2 : Saturate  Commented=on  UpperLimit=20  LowerLimit=-20
  v_as : Outport
  v_bs : Outport  Port=2
  v_cs : Outport  Port=3
  wires:
  v_as*/1 -> Gain/1
  v_bs*/1 -> Gain1/1
  v_cs*/1 -> Gain2/1
  Gain/1 -> v_as/1
  Gain1/1 -> v_bs/1
  Gain2/1 -> v_cs/1

== system main2/5.2.1 ids = 2/Modulador de corriente ==
  I_qs* : Inport
  I_ds* : Inport  Port=2
  I_0s* : Inport  Port=3
  i_qs : Inport  Port=4
  i_ds : Inport  Port=5
  i_0s : Inport  Port=6
  Gain : Gain  Gain=5000*L_q
  Gain1 : Gain  Gain=5000*L_d
  Gain2 : Gain  Gain=5000*L_ls
  Sum : Sum  Inputs=+-
  Sum1 : Sum  Inputs=+-
  Sum2 : Sum  Inputs=+-
  v_qs* : Outport
  v_ds* : Outport  Port=2
  v_0s* : Outport  Port=3
  wires:
  Sum2/1 -> Gain2/1
  Sum1/1 -> Gain1/1
  Sum/1 -> Gain/1
  I_qs*/1 -> Sum/1
  i_qs/1 -> Sum/2
  I_ds*/1 -> Sum1/1
  i_ds/1 -> Sum1/2
  I_0s*/1 -> Sum2/1
  i_0s/1 -> Sum2/2
  Gain/1 -> v_qs*/1
  Gain2/1 -> v_0s*/1
  Gain1/1 -> v_ds*/1

== system main2/5.2.1 ids = 2/Modulador de torque ==
  Tm* : Inport
  ids : Inport  Port=2
  omega_m : Inport  Port=3
  Constant : Constant  Value=lambda_m
  Divide : Product  Inputs=/*
  Gain : Gain  Gain=b_m + b_l/r^2
  Gain1 : Gain  Gain=2/(3*P_p)
  Gain2 : Gain  Gain=L_d-L_q
  Sum : Sum  Inputs=|++
  Sum1 : Sum  Inputs=++|
  iq* : Outport
  wires:
  omega_m/1 -> Gain/1
  Sum/1 -> Gain1/1
  ids/1 -> Gain2/1
  Gain2/1 -> Sum1/1
  Constant/1 -> Sum1/2
  Sum1/1 -> Divide/1
  Gain/1 -> Sum/2
  Tm*/1 -> Sum/1
  Gain1/1 -> Divide/2
  Divide/1 -> iq*/1

== system main2/5.2.1 ids = 2/Observador de estado reducido ==
  T_m* : Inport
  theta_m : Inport  Port=2
  Gain : Gain  Gain=1/(J_m+(J_l/r^2))
  Gain1 : Gain  Gain=K_e_theta
  Gain2 : Gain  Gain=K_e_omega
  Integrator : Integrator
  Integrator1 : Integrator
  Sum : Sum  Inputs=|++
  Sum1 : Sum  Inputs=|++
  Sum2 : Sum  Inputs=|-+
  omega_m_obs : Outport
  theta_m_obs : Outport  Port=2
  wires:
  T_m*/1 -> Gain/1
  Gain/1 -> Sum/1
  Sum/1 -> Integrator/1
  Integrator1/1 -> theta_m_obs/1, Sum2/1
  Integrator/1 -> Sum1/1
  Sum1/1 -> omega_m_obs/1, Integrator1/1
  theta_m/1 -> Sum2/2
  Gain1/1 -> Sum1/2
  Sum2/1 -> Gain2/1, Gain1/1
  Gain2/1 -> Sum/2

== system main2/5.2.1 ids = 2/Sensores ==
  theta_m : Inport
  T_s : Inport  Port=2
  i_as : Inport  Port=3
  i_bs : Inport  Port=4
  i_cs : Inport  Port=5
  Gain{,1..4} (5 alike) : Gain
  theta_m_medida : Outport
  T_s_medida : Outport  Port=2
  i_as_medida : Outport  Port=3
  i_bs_medida : Outport  Port=4
  i_cs_medida : Outport  Port=5
  wires:
  theta_m/1 -> Gain/1
  T_s/1 -> Gain1/1
  i_as/1 -> Gain2/1
  Gain/1 -> theta_m_medida/1
  Gain1/1 -> T_s_medida/1
  Gain2/1 -> i_as_medida/1
  Gain3/1 -> i_bs_medida/1
  i_bs/1 -> Gain3/1
  i_cs/1 -> Gain4/1
  Gain4/1 -> i_cs_medida/1

== system main2/5.2.1 ids = 2/Setpoint ==
  q1* : Inport
  Derivative : Derivative
  Gain : Gain  Gain=r
  theta_m* : Outport
  omega_m* : Outport  Port=2
  wires:
  q1*/1 -> Gain/1
  Gain/1 -> Derivative/1, theta_m*/1
  Derivative/1 -> omega_m*/1

== system main2/5.2.1 ids = 2/Subsistema físico no lineal  ==
  T_l : Inport
  v_as : Inport  Port=2
  v_bs : Inport  Port=3
  v_cs : Inport  Port=4
  theta_r : Inport  Port=5
  Tº_amb : Inport  Port=6
  Subsistema electromagnético : Subsystem
  Subsistema mecánico completo : Subsystem
  Subsistema térmico : Subsystem
  TD_PARK : MATLAB Function  TreatAsAtomicUnit=on
  TI_PARK : MATLAB Function  TreatAsAtomicUnit=on
  theta_m : Outport
  T_s : Outport  Port=2
  i_as : Outport  Port=3
  i_bs : Outport  Port=4
  i_cs : Outport  Port=5
  omega_m : Outport  Port=6
  T_m : Outport  Port=7
  wires:
  theta_r/1 -> TI_PARK/4(theta_r), TD_PARK/4(theta_r)
  TI_PARK/2(fbs) -> i_bs/1
  v_cs/1 -> TD_PARK/3(fcs)
  v_as/1 -> TD_PARK/1(fas)
  TI_PARK/3(fcs) -> i_cs/1
  v_bs/1 -> TD_PARK/2(fbs)
  TI_PARK/1(fas) -> i_as/1
  TD_PARK/1(fqs) -> Subsistema electromagnético/1(v_qs^r)
  TD_PARK/2(fds) -> Subsistema electromagnético/2(v_ds^r)
  TD_PARK/3(f0s) -> Subsistema electromagnético/3(v_0s^r)
  Subsistema mecánico completo/2(omega_m(t)) -> Subsistema electromagnético/4(omega_m), omega_m/1
  Subsistema térmico/2(r_s) -> Subsistema electromagnético/5(r_s)
  Subsistema electromagnético/2(i_ds^r) -> Subsistema térmico/2(i_ds^r), TI_PARK/2(fds)
  Subsistema electromagnético/3(i_qs^r) -> Subsistema térmico/1(i_qs^r), TI_PARK/1(fqs)
  Subsistema electromagnético/1(i_0s^r) -> Subsistema térmico/3(i_0s^r), TI_PARK/3(f0s)
  Subsistema electromagnético/4(T_m) -> Subsistema mecánico completo/1(T_m), T_m/1
  T_l/1 -> Subsistema mecánico completo/2(T_l)
  Tº_amb/1 -> Subsistema térmico/4(Tº_amb)
  Subsistema térmico/1(T_s) -> T_s/1
  Subsistema mecánico completo/1(theta_m(t)) -> theta_m/1

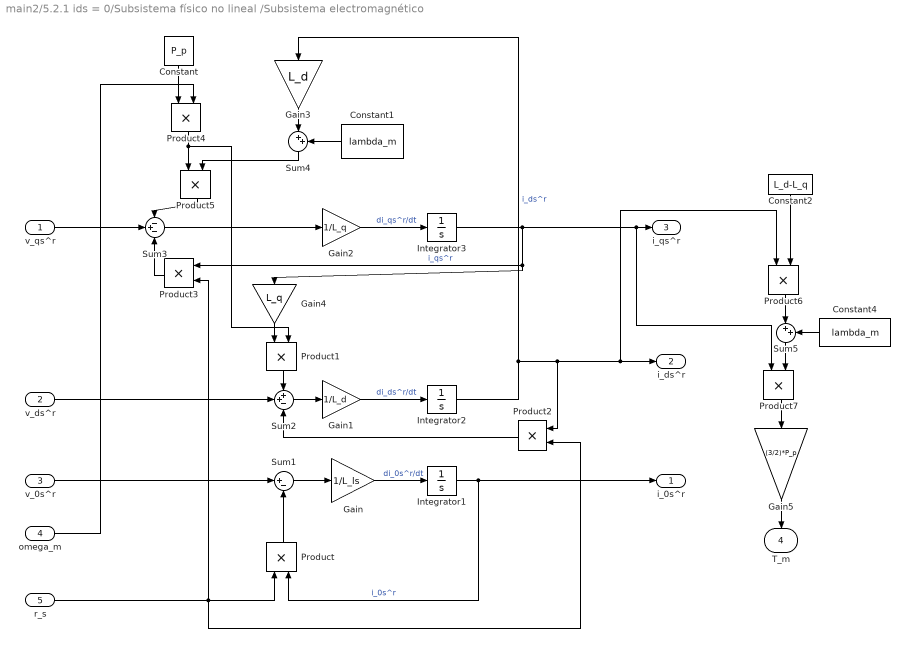
== system main2/5.2.1 ids = 0/Subsistema físico no lineal /Subsistema electromagnético ==
  v_qs^r : Inport
  v_ds^r : Inport  Port=2
  v_0s^r : Inport  Port=3
  omega_m : Inport  Port=4
  r_s : Inport  Port=5
  Constant : Constant  Value=P_p
  Constant1 : Constant  Value=lambda_m
  Constant2 : Constant  Value=L_d-L_q
  Constant4 : Constant  Value=lambda_m
  Gain : Gain  Gain=1/L_ls
  Gain1 : Gain  Gain=1/L_d
  Gain2 : Gain  Gain=1/L_q
  Gain3 : Gain  Gain=L_d
  Gain4 : Gain  Gain=L_q
  Gain5 : Gain  Gain=(3/2)*P_p
  Integrator1 : Integrator
  Integrator2 : Integrator
  Integrator3 : Integrator
  Product{,1..7} (8 alike) : Product
  Sum1 : Sum  Inputs=|+-
  Sum2 : Sum  Inputs=++-
  Sum3 : Sum  Inputs=-+-
  Sum4 : Sum  Inputs=|++
  Sum5 : Sum  Inputs=|++
  i_0s^r : Outport
  i_ds^r : Outport  Port=2
  i_qs^r : Outport  Port=3
  T_m : Outport  Port=4
  wires:
  Constant2/1 -> Product6/2
  Gain5/1 -> T_m/1
  Product5/1 -> Sum3/1
  Product2/1 -> Sum2/3
  Product6/1 -> Sum5/1
  Product1/1 -> Sum2/1
  Gain4/1 -> Product1/1
  Constant4/1 -> Sum5/2
  Sum3/1 -> Gain2/1
  Constant1/1 -> Sum4/2
  Integrator1/1 -> i_0s^r/1, Product/2  "i_0s^r"
  v_ds^r/1 -> Sum2/2
  Product4/1 -> Product1/2, Product5/1
  Sum5/1 -> Product7/2
  Product7/1 -> Gain5/1
  Integrator2/1 -> Gain3/1, Product2/1, Product6/1, i_ds^r/1  "i_ds^r"
  Sum4/1 -> Product5/2
  Product/1 -> Sum1/2
  Integrator3/1 -> Product3/1, Gain4/1, Product7/1, i_qs^r/1  "i_qs^r"
  Product3/1 -> Sum3/3
  Gain/1 -> Integrator1/1  "di_0s^r/dt"
  Gain3/1 -> Sum4/1
  omega_m/1 -> Product4/2
  Constant/1 -> Product4/1
  Sum1/1 -> Gain/1
  r_s/1 -> Product3/2, Product2/2, Product/1
  v_qs^r/1 -> Sum3/2
  Gain2/1 -> Integrator3/1  "di_qs^r/dt"
  v_0s^r/1 -> Sum1/1
  Gain1/1 -> Integrator2/1  "di_ds^r/dt"
  Sum2/1 -> Gain1/1

== system main2/5.2.1 ids = 0/Subsistema físico no lineal /Subsistema mecánico completo ==
  T_m : Inport
  T_l : Inport  Port=2
  Gain : Gain  Gain=b_m +( b_l / (r^2))
  Gain1 : Gain  Gain=1/r
  Gain2 : Gain  Gain=1/(J_m + J_l / (r^2))
  Sum : Sum  Inputs=-+-
  omega_m(0) = 0 : Integrator
  theta_m(0) = 0 : Integrator
  theta_m(t) : Outport
  omega_m(t) : Outport  Port=2
  wires:
  Gain2/1 -> omega_m(0) = 0/1  "domega_m(t)/dt"
  Gain1/1 -> Sum/1
  theta_m(0) = 0/1 -> theta_m(t)/1  "theta_m(t)"
  omega_m(0) = 0/1 -> omega_m(t)/1, Gain/1, theta_m(0) = 0/1  "omega_m(t)"
  Sum/1 -> Gain2/1
  Gain/1 -> Sum/3
  T_l/1 -> Gain1/1
  T_m/1 -> Sum/2

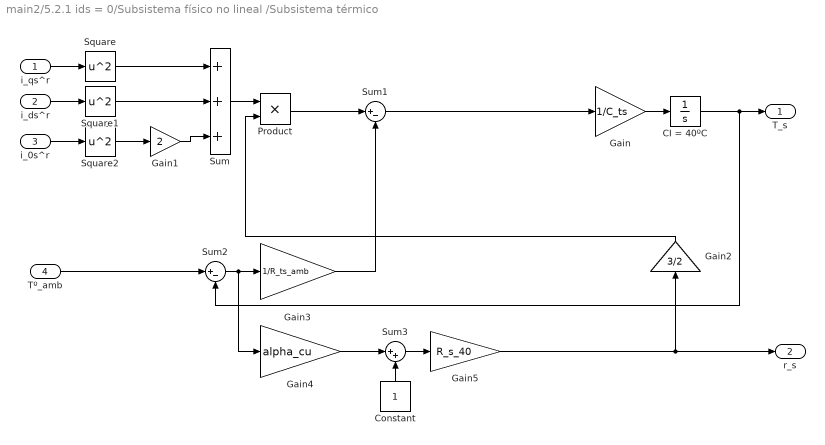
== system main2/5.2.1 ids = 0/Subsistema físico no lineal /Subsistema térmico ==
  i_qs^r : Inport
  i_ds^r : Inport  Port=2
  i_0s^r : Inport  Port=3
  Tº_amb : Inport  Port=4
  CI = 40ºC : Integrator  InitialCondition=40
  Constant : Constant
  Gain : Gain  Gain=1/C_ts
  Gain1 : Gain  Gain=2
  Gain2 : Gain  Gain=3/2
  Gain3 : Gain  Gain=1/R_ts_amb
  Gain4 : Gain  Gain=alpha_cu
  Gain5 : Gain  Gain=R_s_40
  Product : Product
  Square : Math  Operator=square
  Square1 : Math  Operator=square
  Square2 : Math  Operator=square
  Sum : Sum  Inputs=+++
  Sum1 : Sum  Inputs=|+-
  Sum2 : Sum  Inputs=|+-
  Sum3 : Sum  Inputs=|++
  T_s : Outport
  r_s : Outport  Port=2
  wires:
  CI = 40ºC/1 -> Sum2/2, T_s/1
  Gain/1 -> CI = 40ºC/1
  Sum1/1 -> Gain/1
  i_qs^r/1 -> Square/1
  i_ds^r/1 -> Square1/1
  i_0s^r/1 -> Square2/1
  Square2/1 -> Gain1/1
  Square/1 -> Sum/1
  Square1/1 -> Sum/2
  Gain1/1 -> Sum/3
  Gain5/1 -> r_s/1, Gain2/1
  Gain2/1 -> Product/2
  Sum/1 -> Product/1
  Product/1 -> Sum1/1
  Tº_amb/1 -> Sum2/1
  Sum2/1 -> Gain4/1, Gain3/1
  Gain3/1 -> Sum1/2
  Gain4/1 -> Sum3/1
  Constant/1 -> Sum3/2
  Sum3/1 -> Gain5/1

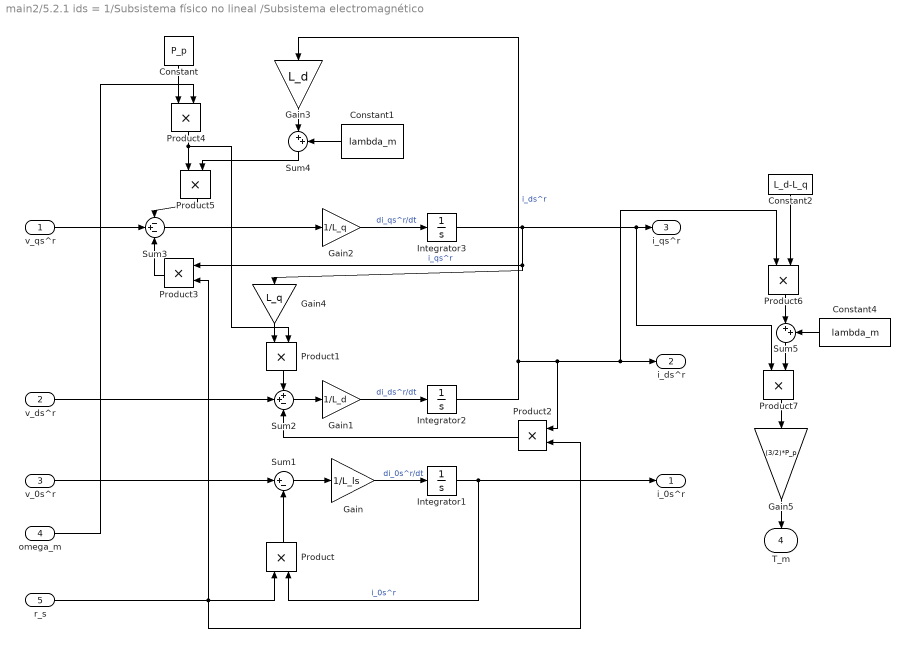
== system main2/5.2.1 ids = 1/Subsistema físico no lineal /Subsistema electromagnético ==
  v_qs^r : Inport
  v_ds^r : Inport  Port=2
  v_0s^r : Inport  Port=3
  omega_m : Inport  Port=4
  r_s : Inport  Port=5
  Constant : Constant  Value=P_p
  Constant1 : Constant  Value=lambda_m
  Constant2 : Constant  Value=L_d-L_q
  Constant4 : Constant  Value=lambda_m
  Gain : Gain  Gain=1/L_ls
  Gain1 : Gain  Gain=1/L_d
  Gain2 : Gain  Gain=1/L_q
  Gain3 : Gain  Gain=L_d
  Gain4 : Gain  Gain=L_q
  Gain5 : Gain  Gain=(3/2)*P_p
  Integrator1 : Integrator
  Integrator2 : Integrator
  Integrator3 : Integrator
  Product{,1..7} (8 alike) : Product
  Sum1 : Sum  Inputs=|+-
  Sum2 : Sum  Inputs=++-
  Sum3 : Sum  Inputs=-+-
  Sum4 : Sum  Inputs=|++
  Sum5 : Sum  Inputs=|++
  i_0s^r : Outport
  i_ds^r : Outport  Port=2
  i_qs^r : Outport  Port=3
  T_m : Outport  Port=4
  wires:
  Constant2/1 -> Product6/2
  Gain5/1 -> T_m/1
  Product5/1 -> Sum3/1
  Product2/1 -> Sum2/3
  Product6/1 -> Sum5/1
  Product1/1 -> Sum2/1
  Gain4/1 -> Product1/1
  Constant4/1 -> Sum5/2
  Sum3/1 -> Gain2/1
  Constant1/1 -> Sum4/2
  Integrator1/1 -> i_0s^r/1, Product/2  "i_0s^r"
  v_ds^r/1 -> Sum2/2
  Product4/1 -> Product1/2, Product5/1
  Sum5/1 -> Product7/2
  Product7/1 -> Gain5/1
  Integrator2/1 -> Gain3/1, Product2/1, Product6/1, i_ds^r/1  "i_ds^r"
  Sum4/1 -> Product5/2
  Product/1 -> Sum1/2
  Integrator3/1 -> Product3/1, Gain4/1, Product7/1, i_qs^r/1  "i_qs^r"
  Product3/1 -> Sum3/3
  Gain/1 -> Integrator1/1  "di_0s^r/dt"
  Gain3/1 -> Sum4/1
  omega_m/1 -> Product4/2
  Constant/1 -> Product4/1
  Sum1/1 -> Gain/1
  r_s/1 -> Product3/2, Product2/2, Product/1
  v_qs^r/1 -> Sum3/2
  Gain2/1 -> Integrator3/1  "di_qs^r/dt"
  v_0s^r/1 -> Sum1/1
  Gain1/1 -> Integrator2/1  "di_ds^r/dt"
  Sum2/1 -> Gain1/1

== system main2/5.2.1 ids = 1/Subsistema físico no lineal /Subsistema mecánico completo ==
  T_m : Inport
  T_l : Inport  Port=2
  Gain : Gain  Gain=b_m +( b_l / (r^2))
  Gain1 : Gain  Gain=1/r
  Gain2 : Gain  Gain=1/(J_m + J_l / (r^2))
  Sum : Sum  Inputs=-+-
  omega_m(0) = 0 : Integrator
  theta_m(0) = 0 : Integrator
  theta_m(t) : Outport
  omega_m(t) : Outport  Port=2
  wires:
  Gain2/1 -> omega_m(0) = 0/1  "domega_m(t)/dt"
  Gain1/1 -> Sum/1
  theta_m(0) = 0/1 -> theta_m(t)/1  "theta_m(t)"
  omega_m(0) = 0/1 -> omega_m(t)/1, Gain/1, theta_m(0) = 0/1  "omega_m(t)"
  Sum/1 -> Gain2/1
  Gain/1 -> Sum/3
  T_l/1 -> Gain1/1
  T_m/1 -> Sum/2

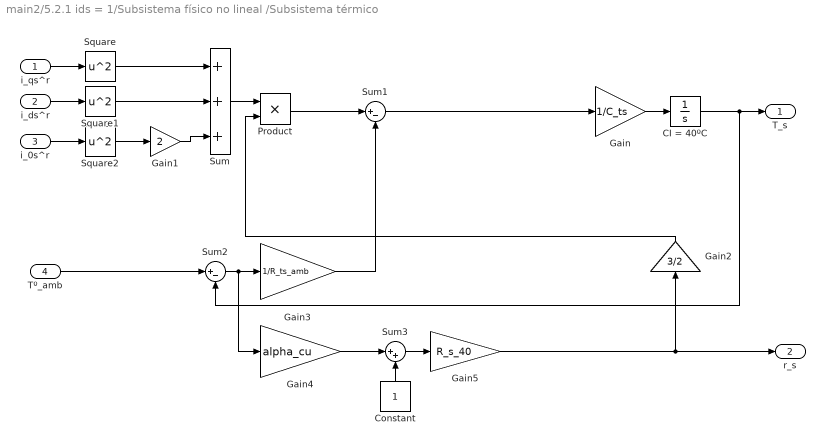
== system main2/5.2.1 ids = 1/Subsistema físico no lineal /Subsistema térmico ==
  i_qs^r : Inport
  i_ds^r : Inport  Port=2
  i_0s^r : Inport  Port=3
  Tº_amb : Inport  Port=4
  CI = 40ºC : Integrator  InitialCondition=40
  Constant : Constant
  Gain : Gain  Gain=1/C_ts
  Gain1 : Gain  Gain=2
  Gain2 : Gain  Gain=3/2
  Gain3 : Gain  Gain=1/R_ts_amb
  Gain4 : Gain  Gain=alpha_cu
  Gain5 : Gain  Gain=R_s_40
  Product : Product
  Square : Math  Operator=square
  Square1 : Math  Operator=square
  Square2 : Math  Operator=square
  Sum : Sum  Inputs=+++
  Sum1 : Sum  Inputs=|+-
  Sum2 : Sum  Inputs=|+-
  Sum3 : Sum  Inputs=|++
  T_s : Outport
  r_s : Outport  Port=2
  wires:
  CI = 40ºC/1 -> Sum2/2, T_s/1
  Gain/1 -> CI = 40ºC/1
  Sum1/1 -> Gain/1
  i_qs^r/1 -> Square/1
  i_ds^r/1 -> Square1/1
  i_0s^r/1 -> Square2/1
  Square2/1 -> Gain1/1
  Square/1 -> Sum/1
  Square1/1 -> Sum/2
  Gain1/1 -> Sum/3
  Gain5/1 -> r_s/1, Gain2/1
  Gain2/1 -> Product/2
  Sum/1 -> Product/1
  Product/1 -> Sum1/1
  Tº_amb/1 -> Sum2/1
  Sum2/1 -> Gain4/1, Gain3/1
  Gain3/1 -> Sum1/2
  Gain4/1 -> Sum3/1
  Constant/1 -> Sum3/2
  Sum3/1 -> Gain5/1

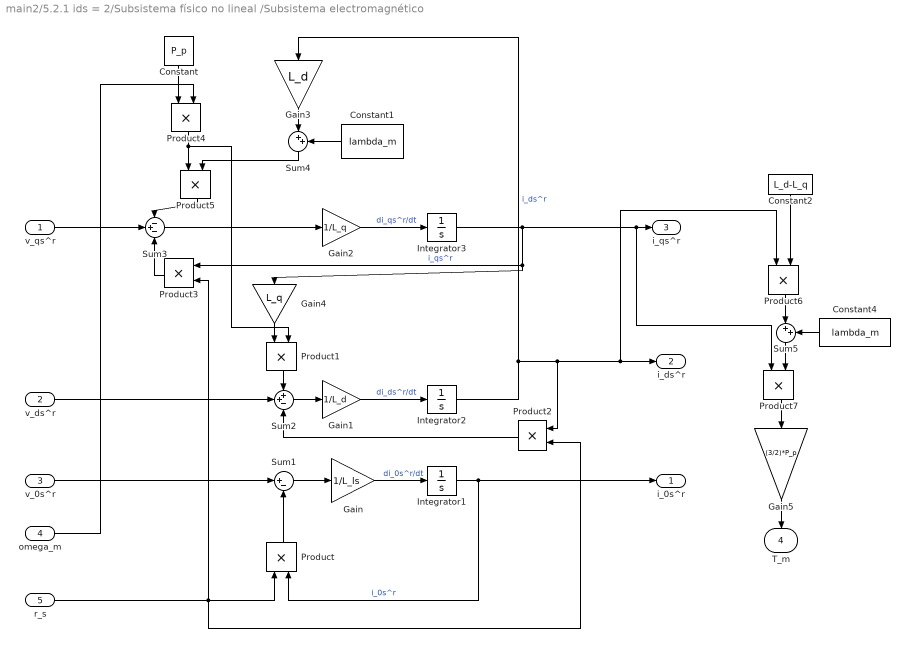
== system main2/5.2.1 ids = 2/Subsistema físico no lineal /Subsistema electromagnético ==
  v_qs^r : Inport
  v_ds^r : Inport  Port=2
  v_0s^r : Inport  Port=3
  omega_m : Inport  Port=4
  r_s : Inport  Port=5
  Constant : Constant  Value=P_p
  Constant1 : Constant  Value=lambda_m
  Constant2 : Constant  Value=L_d-L_q
  Constant4 : Constant  Value=lambda_m
  Gain : Gain  Gain=1/L_ls
  Gain1 : Gain  Gain=1/L_d
  Gain2 : Gain  Gain=1/L_q
  Gain3 : Gain  Gain=L_d
  Gain4 : Gain  Gain=L_q
  Gain5 : Gain  Gain=(3/2)*P_p
  Integrator1 : Integrator
  Integrator2 : Integrator
  Integrator3 : Integrator
  Product{,1..7} (8 alike) : Product
  Sum1 : Sum  Inputs=|+-
  Sum2 : Sum  Inputs=++-
  Sum3 : Sum  Inputs=-+-
  Sum4 : Sum  Inputs=|++
  Sum5 : Sum  Inputs=|++
  i_0s^r : Outport
  i_ds^r : Outport  Port=2
  i_qs^r : Outport  Port=3
  T_m : Outport  Port=4
  wires:
  Constant2/1 -> Product6/2
  Gain5/1 -> T_m/1
  Product5/1 -> Sum3/1
  Product2/1 -> Sum2/3
  Product6/1 -> Sum5/1
  Product1/1 -> Sum2/1
  Gain4/1 -> Product1/1
  Constant4/1 -> Sum5/2
  Sum3/1 -> Gain2/1
  Constant1/1 -> Sum4/2
  Integrator1/1 -> i_0s^r/1, Product/2  "i_0s^r"
  v_ds^r/1 -> Sum2/2
  Product4/1 -> Product1/2, Product5/1
  Sum5/1 -> Product7/2
  Product7/1 -> Gain5/1
  Integrator2/1 -> Gain3/1, Product2/1, Product6/1, i_ds^r/1  "i_ds^r"
  Sum4/1 -> Product5/2
  Product/1 -> Sum1/2
  Integrator3/1 -> Product3/1, Gain4/1, Product7/1, i_qs^r/1  "i_qs^r"
  Product3/1 -> Sum3/3
  Gain/1 -> Integrator1/1  "di_0s^r/dt"
  Gain3/1 -> Sum4/1
  omega_m/1 -> Product4/2
  Constant/1 -> Product4/1
  Sum1/1 -> Gain/1
  r_s/1 -> Product3/2, Product2/2, Product/1
  v_qs^r/1 -> Sum3/2
  Gain2/1 -> Integrator3/1  "di_qs^r/dt"
  v_0s^r/1 -> Sum1/1
  Gain1/1 -> Integrator2/1  "di_ds^r/dt"
  Sum2/1 -> Gain1/1

== system main2/5.2.1 ids = 2/Subsistema físico no lineal /Subsistema mecánico completo ==
  T_m : Inport
  T_l : Inport  Port=2
  Gain : Gain  Gain=b_m +( b_l / (r^2))
  Gain1 : Gain  Gain=1/r
  Gain2 : Gain  Gain=1/(J_m + J_l / (r^2))
  Sum : Sum  Inputs=-+-
  omega_m(0) = 0 : Integrator
  theta_m(0) = 0 : Integrator
  theta_m(t) : Outport
  omega_m(t) : Outport  Port=2
  wires:
  Gain2/1 -> omega_m(0) = 0/1  "domega_m(t)/dt"
  Gain1/1 -> Sum/1
  theta_m(0) = 0/1 -> theta_m(t)/1  "theta_m(t)"
  omega_m(0) = 0/1 -> omega_m(t)/1, Gain/1, theta_m(0) = 0/1  "omega_m(t)"
  Sum/1 -> Gain2/1
  Gain/1 -> Sum/3
  T_l/1 -> Gain1/1
  T_m/1 -> Sum/2

== system main2/5.2.1 ids = 2/Subsistema físico no lineal /Subsistema térmico ==
  i_qs^r : Inport
  i_ds^r : Inport  Port=2
  i_0s^r : Inport  Port=3
  Tº_amb : Inport  Port=4
  CI = 40ºC : Integrator  InitialCondition=40
  Constant : Constant
  Gain : Gain  Gain=1/C_ts
  Gain1 : Gain  Gain=2
  Gain2 : Gain  Gain=3/2
  Gain3 : Gain  Gain=1/R_ts_amb
  Gain4 : Gain  Gain=alpha_cu
  Gain5 : Gain  Gain=R_s_40
  Product : Product
  Square : Math  Operator=square
  Square1 : Math  Operator=square
  Square2 : Math  Operator=square
  Sum : Sum  Inputs=+++
  Sum1 : Sum  Inputs=|+-
  Sum2 : Sum  Inputs=|+-
  Sum3 : Sum  Inputs=|++
  T_s : Outport
  r_s : Outport  Port=2
  wires:
  CI = 40ºC/1 -> Sum2/2, T_s/1
  Gain/1 -> CI = 40ºC/1
  Sum1/1 -> Gain/1
  i_qs^r/1 -> Square/1
  i_ds^r/1 -> Square1/1
  i_0s^r/1 -> Square2/1
  Square2/1 -> Gain1/1
  Square/1 -> Sum/1
  Square1/1 -> Sum/2
  Gain1/1 -> Sum/3
  Gain5/1 -> r_s/1, Gain2/1
  Gain2/1 -> Product/2
  Sum/1 -> Product/1
  Product/1 -> Sum1/1
  Tº_amb/1 -> Sum2/1
  Sum2/1 -> Gain4/1, Gain3/1
  Gain3/1 -> Sum1/2
  Gain4/1 -> Sum3/1
  Constant/1 -> Sum3/2
  Sum3/1 -> Gain5/1

== matlab function main2/5.2.1 ids = 0/TI_PARK1 ==
  data: fqs input; fas output; fds input; f0s input; theta_r input; fbs output; fcs output
function [fas, fbs, fcs] = TI_PARK(fqs, fds, f0s , theta_r)

    fqd0s = [fqs; fds; f0s];

    Ks = [cos(theta_r)         sin(theta_r)             1
          cos(theta_r - 2*pi/3) sin(theta_r - 2*pi/3)    1
          cos(theta_r + 2*pi/3) sin(theta_r + 2*pi/3)    1];

    fabcs = Ks * fqd0s;

    fas = fabcs(1);
    fbs = fabcs(2);
    fcs = fabcs(3);

end

== matlab function main2/5.2.1 ids = 0/Subsistema físico no lineal /TD_PARK ==
  data: fas input; fqs output; fbs input; fcs input; theta_r input; fds output; f0s output
function [fqs, fds, f0s] = TD_PARK(fas, fbs, fcs, theta_r)

    fabcs = [fas; fbs; fcs];

    Ks = 2/3*[cos(theta_r) cos(theta_r - 2*pi/3) cos(theta_r + 2*pi/3)
          sin(theta_r) sin(theta_r - 2*pi/3) sin(theta_r + 2*pi/3) 
          1/2          1/2                   1/2];

    fqd0s = Ks * fabcs;

    fqs = fqd0s(1);
    fds = fqd0s(2);
    f0s = fqd0s(3);

end
